simulink model "example_plant"  (R2022b)
settings: Solver=VariableStepAuto  StartTime=0.0  StopTime=10.0  RelTol=1e-3
undefined symbols (not defined in the file or in its folder): Earth, WGS84
libraries: aerolib6dof2 x1
settings Model: DataDictionary=uorb_msg.sldd  Creator=zhanfuyu  LastModifiedBy=zhanfuyu

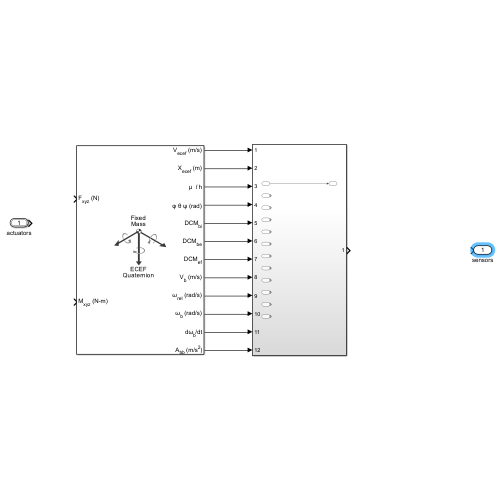
[thumbnail: Simulink's stored preview of the top-level diagram]
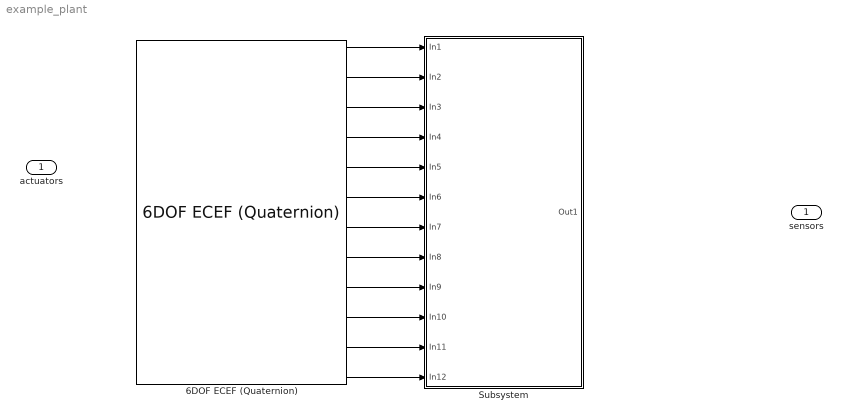
== system example_plant ==
  actuators : Inport  OutDataTypeStr=Bus: actuator_outputs_s
  6DOF ECEF (Quaternion) : aerolib6dof2/6DOF ECEF (Quaternion)  units=Metric (MKS)  mtype=Fixed  xg_0=[0 0 0]  Vm_0=[0 0 0]  eul_0=[0 0 0]  pm_0=[0 0 0]  mass_0=1.0  mass_e=0.5  mass_f=2.0  inertia=eye(3)  inertia_e=eye(3)  inertia_f=2*eye(3)  vre_flag=on  abi_flag=off  ptype=Earth (WGS84)  R=6378137  F=1/298.257223563  w_E=7292115e-11  angle_in=Internal  LG0=0  quat_statename=''  pm_statename=''  Vm_statename=''  posECEF_statename=''  posECI_statename=''  LG_statename=''  mass_statename=''
  Subsystem : Subsystem
  sensors : Outport
  wires:
  6DOF ECEF (Quaternion)/1 -> Subsystem/1(In1)
  6DOF ECEF (Quaternion)/2 -> Subsystem/2(In2)
  6DOF ECEF (Quaternion)/3 -> Subsystem/3(In3)
  6DOF ECEF (Quaternion)/4 -> Subsystem/4(In4)
  6DOF ECEF (Quaternion)/5 -> Subsystem/5(In5)
  6DOF ECEF (Quaternion)/6 -> Subsystem/6(In6)
  6DOF ECEF (Quaternion)/7 -> Subsystem/7(In7)
  6DOF ECEF (Quaternion)/8 -> Subsystem/8(In8)
  6DOF ECEF (Quaternion)/9 -> Subsystem/9(In9)
  6DOF ECEF (Quaternion)/10 -> Subsystem/10(In10)
  6DOF ECEF (Quaternion)/11 -> Subsystem/11(In11)
  6DOF ECEF (Quaternion)/12 -> Subsystem/12(In12)

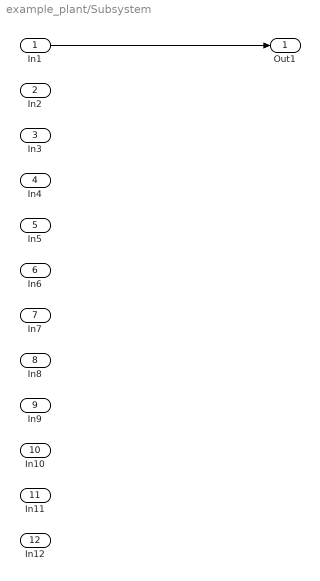
== system example_plant/Subsystem ==
  In1 : Inport
  In2 : Inport  Port=2
  In3 : Inport  Port=3
  In4 : Inport  Port=4
  In5 : Inport  Port=5
  In6 : Inport  Port=6
  In7 : Inport  Port=7
  In8 : Inport  Port=8
  In9 : Inport  Port=9
  In10 : Inport  Port=10
  In11 : Inport  Port=11
  In12 : Inport  Port=12
  Out1 : Outport
  wires:
  In1/1 -> Out1/1
